simulink model "mbdt_autosar_system"  (R2019a)
settings: Solver=FixedStepDiscrete  StartTime=0.0  StopTime=1.5  FixedStep=0.005  RelTol=1e-3  EnableMultiTasking=on
InitFcn:
  | mbd_s32k_as_consistency_checks(bdroot(gcs));
model workspace (MAT data in the model file):
  HBridgeCmd_LkupTbl = Simulink.LookupTable
  HBridgeCmd_LkupTbl.Table = Simulink.lookuptable.Table
  HBridgeCmd_LkupTbl.Table.Value = [-2048 -1843 -1638 -1434 -1229 -1024 -819 -614 -410 -205 0 205 410 614 819 1024 1229 1434 1638 1843 2048]
  HBridgeCmd_LkupTbl.Table.Dimensions = [1 21]
  HBridgeCmd_LkupTbl.Table.DataType = 'int16'
  HBridgeCmd_LkupTbl.Table.FieldName = 'Table'
  HBridgeCmd_LkupTbl.Breakpoints = Simulink.lookuptable.Breakpoint
  HBridgeCmd_LkupTbl.Breakpoints.Value = [-100 -90 -80 -70 -60 -50 -40 -30 -20 -10 0 10 20 30 40 50 60 70 80 90 100]
  HBridgeCmd_LkupTbl.Breakpoints.TunableSizeName = 'N1'
  HBridgeCmd_LkupTbl.Breakpoints.Dimensions = [1 21]
  HBridgeCmd_LkupTbl.Breakpoints.DataType = 'single'
  HBridgeCmd_LkupTbl.Breakpoints.FieldName = 'BP1'
  HBridgeCmd_LkupTbl.SupportTunableSize = 0
  HBridgeCmd_LkupTbl.StructTypeInfo = Simulink.lookuptable.StructTypeInfo
  HBridgeCmd_LkupTbl.StructTypeInfo.Name = 'MyStruct_Actuator'
  HBridgeCmd_LkupTbl.StructTypeInfo.DataScope = 'Auto'
  SetpointPercent_LkupTbl = Simulink.LookupTable
  SetpointPercent_LkupTbl.Table = Simulink.lookuptable.Table
  SetpointPercent_LkupTbl.Table.Value = [0 10 20 30 40 50 60 70 80 90 100]
  SetpointPercent_LkupTbl.Table.Dimensions = [1 11]
  SetpointPercent_LkupTbl.Table.DataType = 'single'
  SetpointPercent_LkupTbl.Table.FieldName = 'Table'
  SetpointPercent_LkupTbl.Breakpoints = Simulink.lookuptable.Breakpoint
  SetpointPercent_LkupTbl.Breakpoints.Value = [170 251.5 333 414.5 496 577.5 659 740.5 822 903.5 985]
  SetpointPercent_LkupTbl.Breakpoints.TunableSizeName = 'N1'
  SetpointPercent_LkupTbl.Breakpoints.Dimensions = [1 11]
  SetpointPercent_LkupTbl.Breakpoints.DataType = 'single'
  SetpointPercent_LkupTbl.Breakpoints.FieldName = 'BP1'
  SetpointPercent_LkupTbl.SupportTunableSize = 0
  SetpointPercent_LkupTbl.StructTypeInfo = Simulink.lookuptable.StructTypeInfo
  SetpointPercent_LkupTbl.StructTypeInfo.Name = 'MyStruct'
  SetpointPercent_LkupTbl.StructTypeInfo.DataScope = 'Auto'
  TPSPercent_LkupTbl = Simulink.LookupTable
  TPSPercent_LkupTbl.Table = Simulink.lookuptable.Table
  TPSPercent_LkupTbl.Table.Value = [0 10 20 30 40 50 60 70 80 90 100]
  TPSPercent_LkupTbl.Table.Dimensions = [1 11]
  TPSPercent_LkupTbl.Table.DataType = 'single'
  TPSPercent_LkupTbl.Table.FieldName = 'Table'
  TPSPercent_LkupTbl.Breakpoints = Simulink.lookuptable.Breakpoint
  TPSPercent_LkupTbl.Breakpoints.Value = [170 249.600006104 329.200012207 408.799987793 488.399993896 568 647.599975586 727.200012207 806.799987793 886.400024414 966]
  TPSPercent_LkupTbl.Breakpoints.TunableSizeName = 'N1'
  TPSPercent_LkupTbl.Breakpoints.Dimensions = [1 11]
  TPSPercent_LkupTbl.Breakpoints.DataType = 'single'
  TPSPercent_LkupTbl.Breakpoints.FieldName = 'BP1'
  TPSPercent_LkupTbl.SupportTunableSize = 0
  TPSPercent_LkupTbl.StructTypeInfo = Simulink.lookuptable.StructTypeInfo
  TPSPercent_LkupTbl.StructTypeInfo.Name = 'MyStruct'
  TPSPercent_LkupTbl.StructTypeInfo.DataScope = 'Auto'
  TPSPrimaryPercent_LkupTbl = Simulink.LookupTable
  TPSPrimaryPercent_LkupTbl.Table = Simulink.lookuptable.Table
  TPSPrimaryPercent_LkupTbl.Table.Value = [0 10 20 30 40 50 60 70 80 90 100]
  TPSPrimaryPercent_LkupTbl.Table.Dimensions = [1 11]
  TPSPrimaryPercent_LkupTbl.Table.DataType = 'single'
  TPSPrimaryPercent_LkupTbl.Table.FieldName = 'Table'
  TPSPrimaryPercent_LkupTbl.Breakpoints = Simulink.lookuptable.Breakpoint
  TPSPrimaryPercent_LkupTbl.Breakpoints.Value = [170 249.600006104 329.200012207 408.799987793 488.399993896 568 647.599975586 727.200012207 806.799987793 886.400024414 966]
  TPSPrimaryPercent_LkupTbl.Breakpoints.TunableSizeName = 'N1'
  TPSPrimaryPercent_LkupTbl.Breakpoints.Dimensions = [1 11]
  TPSPrimaryPercent_LkupTbl.Breakpoints.DataType = 'single'
  TPSPrimaryPercent_LkupTbl.Breakpoints.FieldName = 'BP1'
  TPSPrimaryPercent_LkupTbl.SupportTunableSize = 0
  TPSPrimaryPercent_LkupTbl.StructTypeInfo = Simulink.lookuptable.StructTypeInfo
  TPSPrimaryPercent_LkupTbl.StructTypeInfo.Name = 'MyStruct'
  TPSPrimaryPercent_LkupTbl.StructTypeInfo.DataScope = 'Auto'
  TPSSecondaryPercent_LkupTbl = Simulink.LookupTable
  TPSSecondaryPercent_LkupTbl.Table = Simulink.lookuptable.Table
  TPSSecondaryPercent_LkupTbl.Table.Value = [100 90 80 70 60 50 40 30 20 10 0]
  TPSSecondaryPercent_LkupTbl.Table.Dimensions = [1 11]
  TPSSecondaryPercent_LkupTbl.Table.DataType = 'single'
  TPSSecondaryPercent_LkupTbl.Table.FieldName = 'Table'
  TPSSecondaryPercent_LkupTbl.Breakpoints = Simulink.lookuptable.Breakpoint
  TPSSecondaryPercent_LkupTbl.Breakpoints.Value = [170 249.600006104 329.200012207 408.799987793 488.399993896 568 647.599975586 727.200012207 806.799987793 886.400024414 966]
  TPSSecondaryPercent_LkupTbl.Breakpoints.TunableSizeName = 'N1'
  TPSSecondaryPercent_LkupTbl.Breakpoints.Dimensions = [1 11]
  TPSSecondaryPercent_LkupTbl.Breakpoints.DataType = 'single'
  TPSSecondaryPercent_LkupTbl.Breakpoints.FieldName = 'BP1'
  TPSSecondaryPercent_LkupTbl.SupportTunableSize = 0
  TPSSecondaryPercent_LkupTbl.StructTypeInfo = Simulink.lookuptable.StructTypeInfo
  TPSSecondaryPercent_LkupTbl.StructTypeInfo.Name = 'MyStruct'
  TPSSecondaryPercent_LkupTbl.StructTypeInfo.DataScope = 'Auto'
undefined symbols (not defined in the file or in its folder): LQFP, mthumb, TPSPercentBkpt, TPSPercentTbl
libraries: mbd_s32k_as_ec_toolbox x1, simulink x1
settings Model: OrderedModelArguments=off  Creator=NXP MBDT Team  LastModifiedBy=nxf35401
settings DataIOCC: ExternalInput=off  InitialState=off  SaveOutput=off  SignalLogging=off  SaveTime=off
settings OptimizationCC: DefaultParameterBehavior=Inlined  EnhancedBackFolding=on  PassReuseOutputArgsAs=Individual arguments  ZeroExternalMemoryAtStartup=off  ZeroInternalMemoryAtStartup=off  OptimizeBlockOrder=speed  DifferentSizesBufferReuse=on  OptimizationCustomize=off
settings DebuggingCC: InheritedTsInSrcMsg=none  SingleTaskRateTransMsg=error  ParameterTunabilityLossMsg=error  UnconnectedInputMsg=error  UnconnectedOutputMsg=error  UnconnectedLineMsg=error  UnknownTsInhSupMsg=error  ArithmeticOperatorsInVariantConditions=warning
settings HardwareCC: ProdBitPerPointer=32  ProdBitPerSizeT=32  ProdBitPerPtrDiffT=32  ProdLargestAtomicInteger=Long  ProdLargestAtomicFloat=Double  ProdWordSize=32  ProdHWDeviceType=ARM Compatible->ARM Cortex
settings SFSimCC: MATLABDynamicMemAlloc=off
settings RTWCC: SystemTargetFile=mbd_s32k_as.tlc  MakeCommand=mbd_s32k_as_make_rtw COPY_MDLREF_INCLUDES=0  TemplateMakefile=mbd_s32k_as.tmf  Description=Model Based Design Autosar Toolbox S32K Code Generation Target  GenerateReport=on  IncludeHyperlinkInReport=on  LaunchReport=on  CodeExecutionProfiling=on  CodeProfilingInstrumentation=detailed  GenerateTraceInfo=on  GenerateTraceReport=on  GenerateTraceReportSl=on  GenerateTraceReportSf=on  GenerateTraceReportEml=on
settings CodeAppCC: ForceParamTrailComments=on  IgnoreCustomStorageClasses=off  MaxIdLength=63  OperatorAnnotations=on  SimulinkDataObjDesc=on  SFDataObjDesc=on  InsertBlockDesc=on
settings STFCustomTargetCC: TargetLangStandard=C99 (ISO)  MultiwordLength=256  ParMdlRefBuildCompliant=on  CompOptLevelCompliant=on  IncludeMdlTerminateFcn=off  CombineOutputUpdateFcns=on  SuppressErrorStatus=on  ERTCustomFileBanners=on  SupportAbsoluteTime=off  SupportNonFinite=off  SupportComplex=off  SupportContinuousTime=off  SupportNonInlinedSFcns=off  RemoveResetFunc=on  MATLABClassNameForMDSCustomization=Simulink.SoftwareTarget.ERTCustomization  AutosarCompliant=on  GRTInterface=off  LookupTableObjectStructAxisOrder=2,1,3,4,...  LUTObjectStructOrderEvenSpacing=Size,Table,Breakpoints  SystemTargetFile=mbd_s32k_as.tlc
settings ERTTargetCC: TargetLangStandard=C99 (ISO)  ConcurrentExecutionCompliant=off  IncludeMdlTerminateFcn=off  SuppressErrorStatus=on  SupportAbsoluteTime=off  SupportNonFinite=off  SupportComplex=off  ModelStepFunctionPrototypeControlCompliant=off  CPPClassGenCompliant=off  AutosarCompliant=on  UseToolchainInfoCompliant=off  LookupTableObjectStructAxisOrder=2,1,3,4,...  LUTObjectStructOrderEvenSpacing=Size,Table,Breakpoints  InlinedParameterPlacement=NonHierarchical  ERTSrcFileBannerTemplate=mbd_ert_code_template.cgt  ERTHdrFileBannerTemplate=mbd_ert_code_template.cgt  ERTDataSrcFileTemplate=mbd_ert_code_template.cgt  ERTDataHdrFileTemplate=mbd_ert_code_template.cgt  ERTCustomFileTemplate=example_file_process.tlc

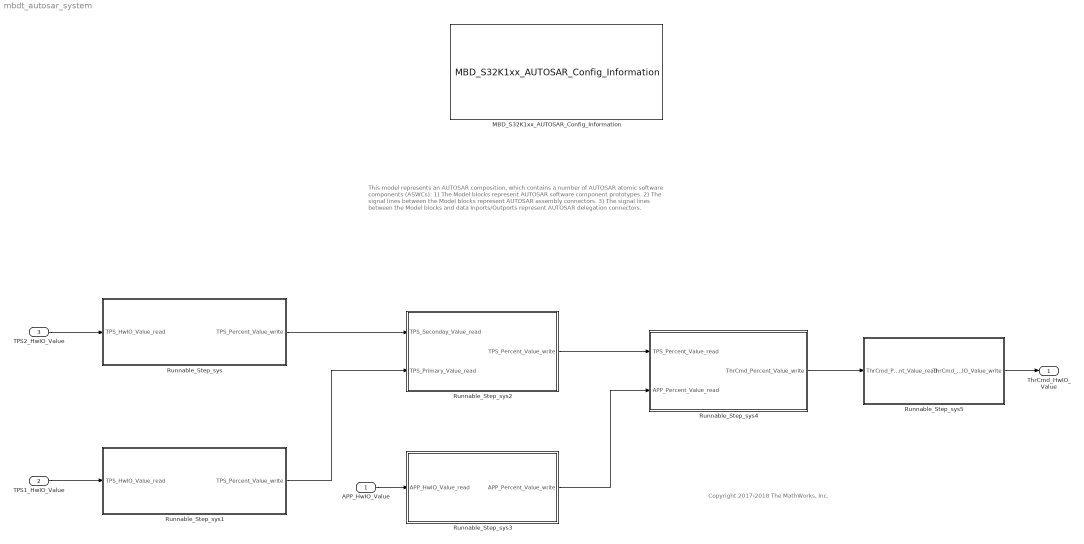
== system mbdt_autosar_system ==
  note: Copyright 2017-2018 The MathWorks, Inc.
  note: This model represents an AUTOSAR composition, which contains a number of AUTOSAR atomic software components (ASWCs):
      | 1) The Model blocks represent AUTOSAR software component prototypes.
      | 2) The signal lines between the Model blocks represent AUTOSAR assembly connectors.
      | 3) The signal lines between the Model blocks and data Inports/Outports represent AUTOSAR delegation connectors.
  APP_HwIO_Value : Inport  OutDataTypeStr=uint16  PortDimensions=1
  TPS1_HwIO_Value : Inport  Port=2  OutDataTypeStr=uint16  PortDimensions=1
  TPS2_HwIO_Value : Inport  Port=3  OutDataTypeStr=uint16  PortDimensions=1
  MBD_S32K1xx_AUTOSAR_Config_Information : mbd_s32k_as_ec_toolbox/MBD_S32K1xx_AUTOSAR_Config_Information  mbdt_ver=0  disp_str=|  config_params=[]  mcu_target_name=S32K116  mcu_target_package=48-LQFP  mcu_target_sram_size=17KB  mcu_system_clock_freq=40  mcu_xtal_freq=External 40  mcu_steptick_timer=LPIT Channel 0  mcu_steptick_prio=3  ds_import_enable=on  target_compiler=GCC  target_memory=FLASH  gcc_target_compile_opts=-mthumb -O1 -g -gstrict-dwarf  gcc_target_assemble_opts=-mthumb -g  gcc_target_link_opts=-mthumb  gcc_target_default_lcf=on  gcc_target_user_lcf=S32K116_17_flash.ld  ghs_target_compile_opts=-mcpu=cortexm0plus -mthumb -fsoft -Ogeneral -Wundef -Wimplicit-int -Wshadow -Wtrigraphs --no_commons --gnu_asm -gnu99 -gdwarf-2 -G  ghs_target_assemble_opts=-mcpu=cortexm0plus -mthumb -fsoft --gnu_asm  ghs_target_link_opts=-mcpu=cortexm0plus -mthumb -fsoft  ghs_target_default_lcf=on  ghs_target_user_lcf=S32K116_17_flash.ld  iar_target_compile_opts=--cpu=Cortex-M4F --thumb --fpu=VFPv4_sp -Ol -e --debug --dlib_config normal  iar_target_assemble_opts=--cpu Cortex-M4F --thumb --fpu VFPv4_sp  iar_target_link_opts=--no_exceptions --vfe --inline  iar_target_default_lcf=on  iar_target_user_lcf=S32K116_17_flash.icf  pil_download_enable=on  rbl_download_enable=off  rbl_start_delay=5000  rbl_download_interface=OpenSDA  rbl_restart_request=off  rbl_com_port=COM29  rbl_com_port_custom=COM1  pil_download_rate=57600  pil_opensda_drive=D: S32K116EVB  pil_opensda_drive_custom=D  pil_uart_instance=0  pil_uart_rx=PTB0: [LPUART0_RX | Receive]  pil_uart_tx=PTB1: [LPUART0_TX | Transmit]  Profile_PcrCheckEnDis=off  ConfigParams_PcrCheckEnDis=off  ModelRef_PcrCheckEnDis=off
      | Target : S32K144-64KB_SRAM
      | Package : 100-pin
      | System clock : 80 MHz
      | XTAL clock : External 8 MHz
      | Compiler : IAR
      | Target Type : FLASH
      | Download Code after build : off
      | Step Tick Interrupt Priority : 15
  Runnable_Step_sys : Subsystem  Priority=3  TreatAsAtomicUnit=on  SystemSampleTime=0.005
  Runnable_Step_sys1 : Subsystem  Priority=2  TreatAsAtomicUnit=on  SystemSampleTime=0.005
  Runnable_Step_sys2 : Subsystem  Priority=4  TreatAsAtomicUnit=on  SystemSampleTime=0.005
  Runnable_Step_sys3 : Subsystem  Priority=5  TreatAsAtomicUnit=on  SystemSampleTime=0.005
  Runnable_Step_sys4 : Subsystem  Priority=6  TreatAsAtomicUnit=on  SystemSampleTime=0.005
  Runnable_Step_sys5 : Subsystem  Priority=6  TreatAsAtomicUnit=on  SystemSampleTime=0.005
  ThrCmd_HwIO_Value : Outport  OutDataTypeStr=int16  PortDimensions=1
  wires:
  Runnable_Step_sys3/1(APP_Percent_Value_write) -> Runnable_Step_sys4/2(APP_Percent_Value_read)
  Runnable_Step_sys/1(TPS_Percent_Value_write) -> Runnable_Step_sys2/1(TPS_Seconday_Value_read)
  Runnable_Step_sys1/1(TPS_Percent_Value_write) -> Runnable_Step_sys2/2(TPS_Primary_Value_read)
  APP_HwIO_Value/1 -> Runnable_Step_sys3/1(APP_HwIO_Value_read)
  TPS2_HwIO_Value/1 -> Runnable_Step_sys/1(TPS_HwIO_Value_read)
  TPS1_HwIO_Value/1 -> Runnable_Step_sys1/1(TPS_HwIO_Value_read)
  Runnable_Step_sys4/1(ThrCmd_Percent_Value_write) -> Runnable_Step_sys5/1(ThrCmd_Percent_Value_read)
  Runnable_Step_sys5/1(ThrCmd_HwIO_Value_write) -> ThrCmd_HwIO_Value/1
  Runnable_Step_sys2/1(TPS_Percent_Value_write) -> Runnable_Step_sys4/1(TPS_Percent_Value_read)

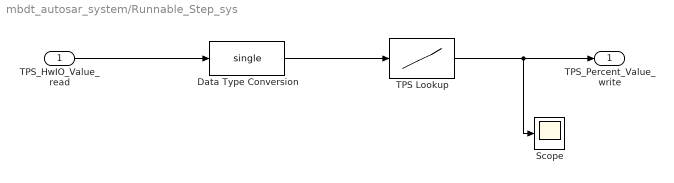
== system mbdt_autosar_system/Runnable_Step_sys ==
  TPS_HwIO_Value_read : Inport
  Data Type Conversion : DataTypeConversion  OutDataTypeStr=single
  Scope : Scope
  TPS Lookup : Lookup_n-D  NumberOfTableDimensions=1  DataSpecification=Lookup table object  LookupTableObject=TPSSecondaryPercent_LkupTbl  BreakpointsForDimension1=TPSPercentBkpt  BreakpointsForDimension1DataTypeStr=single  IndexSearchMethod=Linear search  Table=TPSPercentTbl  TableDataTypeStr=single  ExtrapMethod=Clip  InternalRulePriority=Speed  OutDataTypeStr=single  RndMeth=Simplest  InputSameDT=on
  TPS_Percent_Value_write : Outport
  wires:
  TPS_HwIO_Value_read/1 -> Data Type Conversion/1
  TPS Lookup/1 -> Scope/1, TPS_Percent_Value_write/1
  Data Type Conversion/1 -> TPS Lookup/1

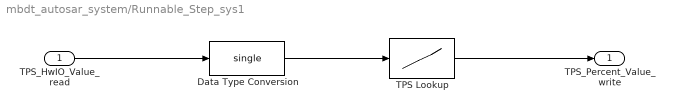
== system mbdt_autosar_system/Runnable_Step_sys1 ==
  TPS_HwIO_Value_read : Inport
  Data Type Conversion : DataTypeConversion  OutDataTypeStr=single
  TPS Lookup : Lookup_n-D  NumberOfTableDimensions=1  DataSpecification=Lookup table object  LookupTableObject=TPSPrimaryPercent_LkupTbl  BreakpointsForDimension1=TPSPercentBkpt  BreakpointsForDimension1DataTypeStr=single  IndexSearchMethod=Linear search  Table=TPSPercentTbl  TableDataTypeStr=single  ExtrapMethod=Clip  InternalRulePriority=Speed  OutDataTypeStr=single  RndMeth=Simplest  InputSameDT=on
  TPS_Percent_Value_write : Outport
  wires:
  TPS_HwIO_Value_read/1 -> Data Type Conversion/1
  TPS Lookup/1 -> TPS_Percent_Value_write/1
  Data Type Conversion/1 -> TPS Lookup/1

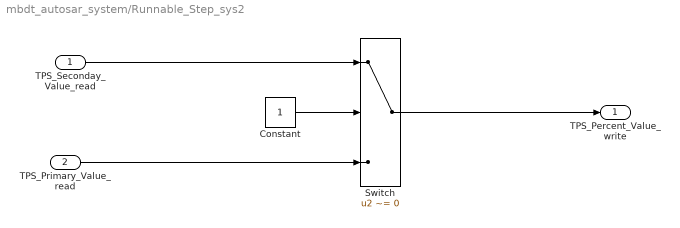
== system mbdt_autosar_system/Runnable_Step_sys2 ==
  TPS_Seconday_Value_read : Inport
  TPS_Primary_Value_read : Inport  Port=2
  Constant : Constant  OutDataTypeStr=boolean
  Switch : Switch  Criteria=u2 ~= 0
  TPS_Percent_Value_write : Outport  PortDimensions=1
  wires:
  TPS_Seconday_Value_read/1 -> Switch/1
  TPS_Primary_Value_read/1 -> Switch/3
  Switch/1 -> TPS_Percent_Value_write/1
  Constant/1 -> Switch/2

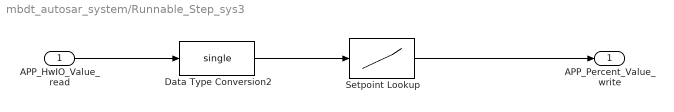
== system mbdt_autosar_system/Runnable_Step_sys3 ==
  APP_HwIO_Value_read : Inport
  Data Type Conversion2 : DataTypeConversion  OutDataTypeStr=single
  Setpoint Lookup : Lookup_n-D  NumberOfTableDimensions=1  DataSpecification=Lookup table object  LookupTableObject=SetpointPercent_LkupTbl  BreakpointsForDimension1=TPSPercentBkpt  BreakpointsForDimension1DataTypeStr=single  IndexSearchMethod=Linear search  Table=TPSPercentTbl  TableDataTypeStr=single  ExtrapMethod=Clip  InternalRulePriority=Speed  OutDataTypeStr=single  RndMeth=Simplest  InputSameDT=on
  APP_Percent_Value_write : Outport
  wires:
  APP_HwIO_Value_read/1 -> Data Type Conversion2/1
  Setpoint Lookup/1 -> APP_Percent_Value_write/1
  Data Type Conversion2/1 -> Setpoint Lookup/1

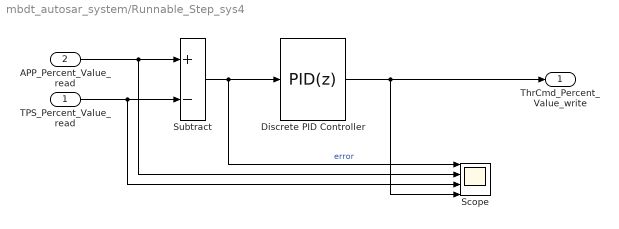
== system mbdt_autosar_system/Runnable_Step_sys4 ==
  TPS_Percent_Value_read : Inport
  APP_Percent_Value_read : Inport  Port=2
  Discrete PID Controller : simulink/Continuous/PID Controller  Controller=PID  Form=Parallel  TimeDomain=Discrete-time  SampleTime=-1  IntegratorMethod=Forward Euler  FilterMethod=Forward Euler  ControllerParametersSource=internal  P=1  I=2  D=0  UseFilter=on  N=100  TunerSelectOption=Transfer Function Based (PID Tuner App)  InitialConditionSource=internal  InitialConditionForIntegrator=0  InitialConditionForFilter=0  DifferentiatorICPrevScaledInput=0  ExternalReset=none  TrackingMode=off  Kt=1  LimitOutput=on  UpperSaturationLimit=100  LowerSaturationLimit=-100  LinearizeAsGain=off  AntiWindupMode=clamping  Kb=1  POutMin=[]  POutMax=[]  IOutMin=[]  IOutMax=[]  DOutMin=[]  DOutMax=[]  NOutMin=[]  NOutMax=[]  SumOutMin=[]  SumOutMax=[]  SaturationOutMin=[]  SaturationOutMax=[]  PParamMin=[]  PParamMax=[]  IParamMin=[]  IParamMax=[]  DParamMin=[]  DParamMax=[]  NParamMin=[]  NParamMax=[]  KbParamMin=[]  KbParamMax=[]  KtParamMin=[]  KtParamMax=[]  KbOutMin=[]  KbOutMax=[]  KtOutMin=[]  KtOutMax=[]  IntegratorOutMin=[]  IntegratorOutMax=[]  FilterOutMin=[]  FilterOutMax=[]  SumI1OutMin=[]  SumI1OutMax=[]  SumI2OutMin=[]  SumI2OutMax=[]  SumI3OutMin=[]  SumI3OutMax=[]  SumI4OutMin=[]  SumI4OutMax=[]  SumDOutMin=[]  SumDOutMax=[]  DifferentiatorOutMin=[]  DifferentiatorOutMax=[]  FilterDiffOutCoefMin=[]  FilterDiffOutCoefMax=[]  ReciprocalOutMin=[]  ReciprocalOutMax=[]  SumDenOutMin=[]  SumDenOutMax=[]  SumNumOutMin=[]  SumNumOutMax=[]  DivideOutMin=[]  DivideOutMax=[]  IntegratorContinuousStateAttributes=''  IntegratorStateMustResolveToSignalObject=off  IntegratorRTWStateStorageClass=Auto  FilterContinuousStateAttributes=''  FilterStateMustResolveToSignalObject=off  FilterRTWStateStorageClass=Auto  ParallelPVariant=InternalParameters  IdealPVariant=Disabled  IVariant=InternalParameters  DVariant=InternalParameters  IntegratorVariant=Discrete  SatVariant=Enabled  AWVariant=DiscClampingParallel  PCopyVariant=Disabled  TRVariant=Disabled  FdbkBlocksVariant=Forward  IdealPFdbkVariant=Disabled  SatFdbkVariant=Disabled  DerivativeFilterVariant=ForwardEulerFilter  NVariant=InternalParameters  NCopyVariant=Disabled  FilterICVariant=InternalICsFilter  IntegratorICVariant=InternalICs  ExternalResetVariant=Disabled  TRSumVariant=Passthrough  SumFdbkVariant=Disabled  SumVariant=Sum_PID
  Scope : Scope  NumInputPorts=4
  Subtract : Sum  Inputs=+-
  ThrCmd_Percent_Value_write : Outport
  wires:
  TPS_Percent_Value_read/1 -> Scope/3, Subtract/2
  APP_Percent_Value_read/1 -> Scope/2, Subtract/1
  Discrete PID Controller/1 -> Scope/4, ThrCmd_Percent_Value_write/1
  Subtract/1 -> Scope/1, Discrete PID Controller/1  "error"

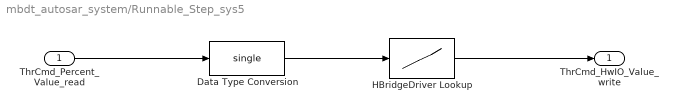
== system mbdt_autosar_system/Runnable_Step_sys5 ==
  ThrCmd_Percent_Value_read : Inport
  Data Type Conversion : DataTypeConversion  OutDataTypeStr=single
  HBridgeDriver Lookup : Lookup_n-D  NumberOfTableDimensions=1  DataSpecification=Lookup table object  LookupTableObject=HBridgeCmd_LkupTbl  BreakpointsForDimension1=TPSPercentBkpt  BreakpointsForDimension1DataTypeStr=single  IndexSearchMethod=Linear search  Table=TPSPercentTbl  TableDataTypeStr=single  InterpMethod=Nearest  InternalRulePriority=Speed  OutDataTypeStr=Inherit: Inherit from 'Table data'  RndMeth=Simplest  InputSameDT=on
  ThrCmd_HwIO_Value_write : Outport
  wires:
  ThrCmd_Percent_Value_read/1 -> Data Type Conversion/1
  HBridgeDriver Lookup/1 -> ThrCmd_HwIO_Value_write/1
  Data Type Conversion/1 -> HBridgeDriver Lookup/1
